simulink model "PID"  (R2022b)
settings: Solver=ode4  StartTime=0.0  StopTime=25  FixedStep=0.02  RelTol=1e-3  EnableMultiTasking=on
undefined symbols (not defined in the file): A3, B3, C2, DiscIntNeverNeededParam, rad, s
libraries: arduinolib x5, aerolibconvert2 x4, simulink_extras x1
settings Model: ExtModeTrigDuration=2  Creator=Ali  LastModifiedBy=Ali
settings SolverCC: AlgebraicLoopSolver=TrustRegion
settings OptimizationCC: EnhancedBackFolding=on  PassReuseOutputArgsAs=Individual arguments  ZeroExternalMemoryAtStartup=off  ZeroInternalMemoryAtStartup=off  MaxStackSize=64  OptimizeBlockOrder=speed  DifferentSizesBufferReuse=on  OptimizationCustomize=off  EfficientTunableParamExpr=on
settings DebuggingCC: ParameterTunabilityLossMsg=error  UnconnectedInputMsg=warning  UnconnectedOutputMsg=warning  UnconnectedLineMsg=warning  SFMachineParentedDataDiag=warning
settings HardwareCC: ProdBitPerInt=16  ProdBitPerPointer=16  ProdBitPerSizeT=16  ProdBitPerPtrDiffT=16  ProdLargestAtomicFloat=None  ProdWordSize=8  ProdHWDeviceType=Atmel->AVR
settings ModelReferenceCC: EnableRefExpFcnMdlSchedulingChecks=on
settings SFSimCC: MATLABDynamicMemAlloc=off
settings RTWCC: Description=Embedded Coder  SystemTargetFile=ert.tlc  HardwareBoard=Arduino Mega 2560  TLCOptions=-aInlineSetEventsForThisBaseRateFcn=TLC_FALSE -aSuppressMultiTaskScheduler=TLC_FALSE -aRateBasedStepFcn=1  TemplateMakefile=ert_default_tmf  Toolchain=Arduino AVR  BuildConfiguration=Faster Runs
settings CodeAppCC: ForceParamTrailComments=on  IgnoreCustomStorageClasses=off  OperatorAnnotations=on  SimulinkDataObjDesc=on  SFDataObjDesc=on  InsertBlockDesc=on
settings ERTTargetCC: SupportContinuousTime=on  SupportVariableSizeSignals=on  ExtModeStaticAllocSize=2048

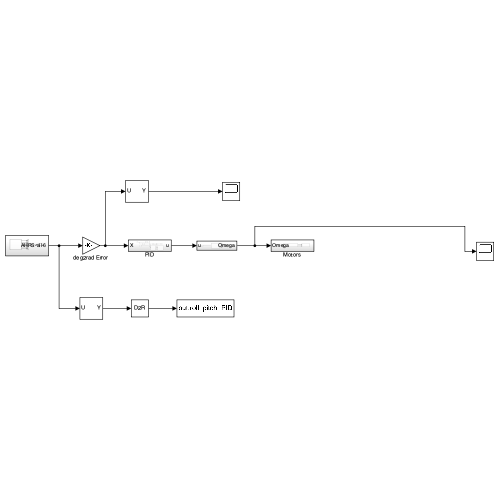
[thumbnail: Simulink's stored preview of the top-level diagram]
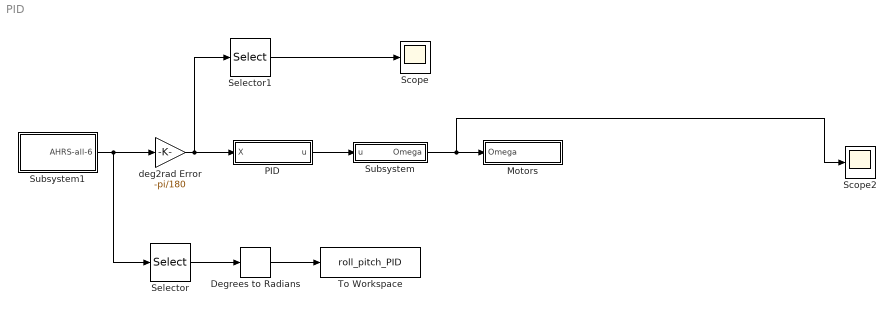
== system PID ==
  Degrees to Radians : simulink_extras/Transformations/Degrees to Radians
  Motors : Subsystem
  PID : Subsystem
  Scope : Scope
  Scope2 : Scope
  Selector : Selector  InputPortWidth=6  IndexOptions=Index vector (dialog)  Indices=[1 2 4 5]  OutputSizes=1
  Selector1 : Selector  InputPortWidth=6  IndexOptions=Index vector (dialog)  Indices=[1 2]  OutputSizes=1
  Subsystem : Subsystem
  Subsystem1 : Subsystem
  To Workspace : ToWorkspace  VariableName=roll_pitch_PID  SampleTime=-1
  deg2rad Error : Gain  Gain=-pi/180
  wires:
  Subsystem/1(Omega) -> Scope2/1, Motors/1(Omega)
  PID/1(u) -> Subsystem/1(u)
  Subsystem1/1(AHRS-all-6) -> Selector/1, deg2rad Error/1
  Selector/1 -> Degrees to Radians/1
  Degrees to Radians/1 -> To Workspace/1
  deg2rad Error/1 -> Selector1/1, PID/1(X)
  Selector1/1 -> Scope/1

== system PID/Motors ==
  Omega : Inport
  Arduino PWM1 : Subsystem  mask{Motor1=8, Motor2=9, Motor3=10, Motor4=11}
      mask prompts: Motor1 "Motor 1 Pin Number"; Motor2 "Motor 2 Pin Number"; Motor3 "Motor 3 Pin Number"; Motor4 "Motor 4 Pin Number"
  Convert To Duty Cycle : Subsystem
  Demux : Demux
  wires:
  Convert To Duty Cycle/4(duty_cycle4 (0-255)) -> Arduino PWM1/4(duty_cycle4 (0-255))
  Demux/4 -> Convert To Duty Cycle/4(Omega_Command4)
  Demux/3 -> Convert To Duty Cycle/3(Omega_Command3)
  Convert To Duty Cycle/2(duty_cycle2 (0-255)) -> Arduino PWM1/2(duty_cycle2 (0-255))
  Convert To Duty Cycle/1(duty_cycle1 (0-255)) -> Arduino PWM1/1(duty_cycle1 (0-255))
  Omega/1 -> Demux/1
  Demux/2 -> Convert To Duty Cycle/2(Omega_Command2)
  Demux/1 -> Convert To Duty Cycle/1(Omega_Command1)
  Convert To Duty Cycle/3(duty_cycle3 (0-255)) -> Arduino PWM1/3(duty_cycle3 (0-255))

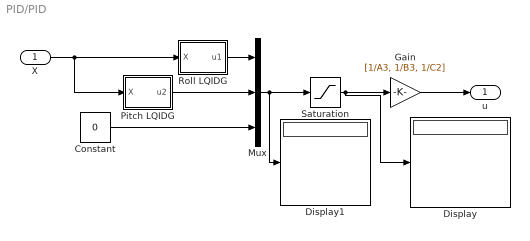
== system PID/PID ==
  X : Inport
  Constant : Constant  Value=0
  Display : Display
  Display1 : Display
  Gain : Gain  Gain=[1/A3, 1/B3, 1/C2]
  Mux : Mux  Inputs=3
  Pitch LQIDG : Subsystem
  Roll LQIDG : Subsystem
  Saturation : Saturate  UpperLimit=12  LowerLimit=-12
  u : Outport
  wires:
  Mux/1 -> Display1/1, Saturation/1
  Gain/1 -> u/1
  Saturation/1 -> Display/1, Gain/1
  Constant/1 -> Mux/3
  Pitch LQIDG/1(u2) -> Mux/2
  X/1 -> Pitch LQIDG/1(X), Roll LQIDG/1(X)
  Roll LQIDG/1(u1) -> Mux/1

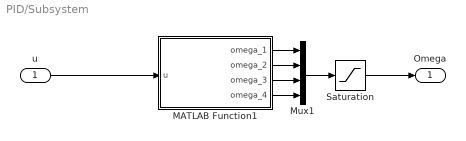
== system PID/Subsystem ==
  u : Inport
  MATLAB Function1 : MATLAB Function  TreatAsAtomicUnit=on
  Mux1 : Mux
  Saturation : Saturate  UpperLimit=6000/60*2*pi  LowerLimit=1000/60*2*pi
  Omega : Outport
  wires:
  MATLAB Function1/1(omega_1) -> Mux1/1
  MATLAB Function1/2(omega_2) -> Mux1/2
  MATLAB Function1/4(omega_4) -> Mux1/4
  Mux1/1 -> Saturation/1
  MATLAB Function1/3(omega_3) -> Mux1/3
  Saturation/1 -> Omega/1
  u/1 -> MATLAB Function1/1(u)

== system PID/Subsystem1 ==
  AHRS : Subsystem
  Mux : Mux  Inputs=6
  AHRS-all-6 : Outport
  wires:
  Mux/1 -> AHRS-all-6/1
  AHRS/4(roll_rate) -> Mux/4
  AHRS/2(theta) -> Mux/2
  AHRS/6(yaw_rate) -> Mux/6
  AHRS/1(phi) -> Mux/1
  AHRS/5(pitch_rate) -> Mux/5
  AHRS/3(psi) -> Mux/3

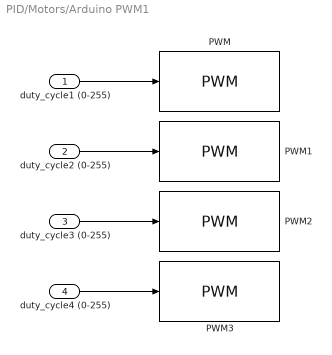
== system PID/Motors/Arduino PWM1 ==
  duty_cycle1 (0-255) : Inport
  duty_cycle2 (0-255) : Inport  Port=2
  duty_cycle3 (0-255) : Inport  Port=3
  duty_cycle4 (0-255) : Inport  Port=4
  PWM : arduinolib/PWM  pinNumber=8  frequencyType=Default  desiredFrequency=490.2  achievableFrequency=490.2
  PWM1 : arduinolib/PWM  pinNumber=9  frequencyType=Default  desiredFrequency=490.2  achievableFrequency=490.2
  PWM2 : arduinolib/PWM  pinNumber=10  frequencyType=Default  desiredFrequency=490.2  achievableFrequency=490.2
  PWM3 : arduinolib/PWM  pinNumber=11  frequencyType=Default  desiredFrequency=490.2  achievableFrequency=490.2
  wires:
  duty_cycle1 (0-255)/1 -> PWM/1
  duty_cycle2 (0-255)/1 -> PWM1/1
  duty_cycle3 (0-255)/1 -> PWM2/1
  duty_cycle4 (0-255)/1 -> PWM3/1

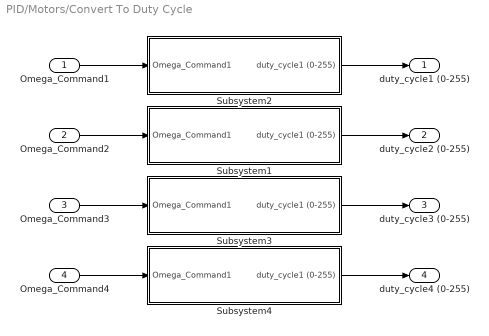
== system PID/Motors/Convert To Duty Cycle ==
  Omega_Command1 : Inport
  Omega_Command2 : Inport  Port=2
  Omega_Command3 : Inport  Port=3
  Omega_Command4 : Inport  Port=4
  Subsystem1 : Subsystem
  Subsystem2 : Subsystem
  Subsystem3 : Subsystem
  Subsystem4 : Subsystem
  duty_cycle1 (0-255) : Outport
  duty_cycle2 (0-255) : Outport  Port=2
  duty_cycle3 (0-255) : Outport  Port=3
  duty_cycle4 (0-255) : Outport  Port=4
  wires:
  Subsystem1/1(duty_cycle1 (0-255)) -> duty_cycle2 (0-255)/1
  Subsystem3/1(duty_cycle1 (0-255)) -> duty_cycle3 (0-255)/1
  Subsystem4/1(duty_cycle1 (0-255)) -> duty_cycle4 (0-255)/1
  Subsystem2/1(duty_cycle1 (0-255)) -> duty_cycle1 (0-255)/1
  Omega_Command1/1 -> Subsystem2/1(Omega_Command1)
  Omega_Command4/1 -> Subsystem4/1(Omega_Command1)
  Omega_Command3/1 -> Subsystem3/1(Omega_Command1)
  Omega_Command2/1 -> Subsystem1/1(Omega_Command1)

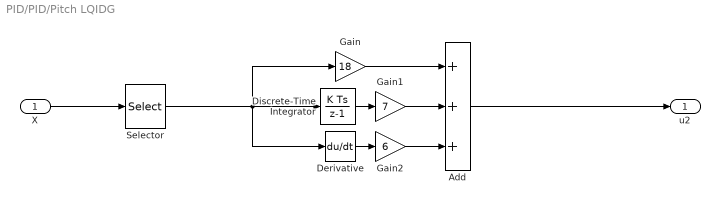
== system PID/PID/Pitch LQIDG ==
  X : Inport
  Add : Sum  Inputs=+++
  Derivative : Derivative
  Discrete-Time Integrator : DiscreteIntegrator  SampleTime=-1  ICPrevOutput=DiscIntNeverNeededParam  ICPrevScaledInput=DiscIntNeverNeededParam
  Gain : Gain  Gain=18
  Gain1 : Gain  Gain=7
  Gain2 : Gain  Gain=6
  Selector : Selector  InputPortWidth=6  IndexOptions=Index vector (dialog)  Indices=[2]  OutputSizes=1
  u2 : Outport
  wires:
  X/1 -> Selector/1
  Selector/1 -> Discrete-Time Integrator/1, Gain/1, Derivative/1
  Gain1/1 -> Add/2
  Gain2/1 -> Add/3
  Discrete-Time Integrator/1 -> Gain1/1
  Derivative/1 -> Gain2/1
  Gain/1 -> Add/1
  Add/1 -> u2/1

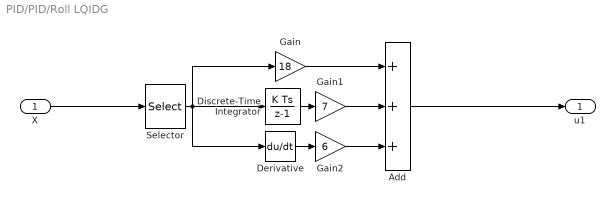
== system PID/PID/Roll LQIDG ==
  X : Inport
  Add : Sum  Inputs=+++
  Derivative : Derivative
  Discrete-Time Integrator : DiscreteIntegrator  SampleTime=-1  ICPrevOutput=DiscIntNeverNeededParam  ICPrevScaledInput=DiscIntNeverNeededParam
  Gain : Gain  Gain=18
  Gain1 : Gain  Gain=7
  Gain2 : Gain  Gain=6
  Selector : Selector  InputPortWidth=6  IndexOptions=Index vector (dialog)  Indices=[1]  OutputSizes=1
  u1 : Outport
  wires:
  X/1 -> Selector/1
  Selector/1 -> Discrete-Time Integrator/1, Derivative/1, Gain/1
  Gain/1 -> Add/1
  Discrete-Time Integrator/1 -> Gain1/1
  Gain1/1 -> Add/2
  Gain2/1 -> Add/3
  Derivative/1 -> Gain2/1
  Add/1 -> u1/1

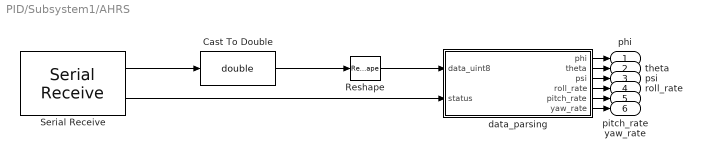
== system PID/Subsystem1/AHRS ==
  Cast To Double : DataTypeConversion  OutDataTypeStr=double  SaturateOnIntegerOverflow=off  RndMeth=Floor
  Reshape : Reshape
  Serial Receive : arduinolib/Serial Receive  isARMArch=off  portNumber=1  DataType=uint8  Datalength=32  SampleTime=0.02  showOutStatus=on  blockPlatform=arduino
  data_parsing : MATLAB Function  TreatAsAtomicUnit=on
  phi : Outport
  theta : Outport  Port=2
  psi : Outport  Port=3
  roll_rate : Outport  Port=4
  pitch_rate : Outport  Port=5
  yaw_rate : Outport  Port=6
  wires:
  data_parsing/2(theta) -> theta/1
  data_parsing/3(psi) -> psi/1
  data_parsing/4(roll_rate) -> roll_rate/1
  Reshape/1 -> data_parsing/1(data_uint8)
  data_parsing/1(phi) -> phi/1
  data_parsing/5(pitch_rate) -> pitch_rate/1
  Serial Receive/2 -> data_parsing/2(status)
  data_parsing/6(yaw_rate) -> yaw_rate/1
  Cast To Double/1 -> Reshape/1
  Serial Receive/1 -> Cast To Double/1

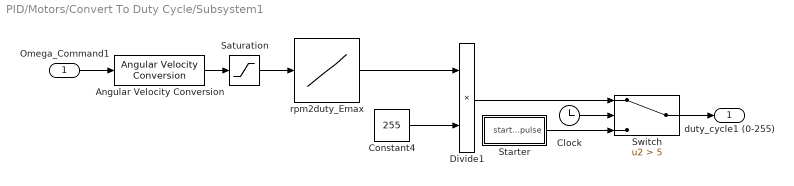
== system PID/Motors/Convert To Duty Cycle/Subsystem1 ==
  Omega_Command1 : Inport
  Angular Velocity Conversion : aerolibconvert2/Angular Velocity Conversion  IU=rad/s  OU=rpm
  Clock : Clock
  Constant4 : Constant  Value=255
  Divide1 : Product  Inputs=**
  Saturation : Saturate  UpperLimit=6000  LowerLimit=1300
  Starter : Subsystem
  Switch : Switch  Criteria=u2 > Threshold  Threshold=5  SaturateOnIntegerOverflow=off  InputSameDT=off
  rpm2duty_Emax : Lookup_n-D  NumberOfTableDimensions=1  BreakpointsForDimension1=|  Table=|  RndMeth=Simplest
      BreakpointsForDimension1=|
      | [1201
      | 2305
      | 3096
      | 3930
      | 4118
      | 4555
      | 5122
      | 5552
      | 5957
      | 6291
      | 6360]
      Table=|
      | [0.5
      | 0.55
      | 0.6
      | 0.65
      | 0.7
      | 0.75
      | 0.8
      | 0.85
      | 0.9
      | 0.95
      | 1]
  duty_cycle1 (0-255) : Outport
  wires:
  Divide1/1 -> Switch/1
  Switch/1 -> duty_cycle1 (0-255)/1
  Clock/1 -> Switch/2
  Starter/1(start_pulse) -> Switch/3
  Angular Velocity Conversion/1 -> Saturation/1
  Constant4/1 -> Divide1/2
  Omega_Command1/1 -> Angular Velocity Conversion/1
  rpm2duty_Emax/1 -> Divide1/1
  Saturation/1 -> rpm2duty_Emax/1

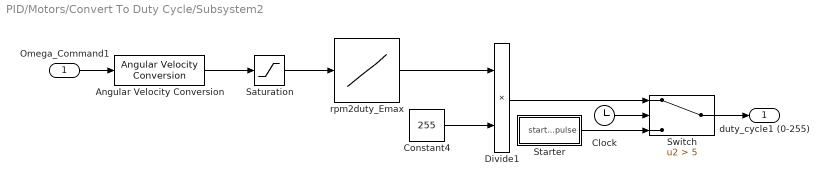
== system PID/Motors/Convert To Duty Cycle/Subsystem2 ==
  Omega_Command1 : Inport
  Angular Velocity Conversion : aerolibconvert2/Angular Velocity Conversion  IU=rad/s  OU=rpm
  Clock : Clock
  Constant4 : Constant  Value=255
  Divide1 : Product  Inputs=**
  Saturation : Saturate  UpperLimit=6000  LowerLimit=1300
  Starter : Subsystem
  Switch : Switch  Criteria=u2 > Threshold  Threshold=5  SaturateOnIntegerOverflow=off  InputSameDT=off
  rpm2duty_Emax : Lookup_n-D  NumberOfTableDimensions=1  BreakpointsForDimension1=|  Table=|  RndMeth=Simplest
      BreakpointsForDimension1=|
      | [1201
      | 2305
      | 3096
      | 3930
      | 4118
      | 4555
      | 5122
      | 5552
      | 5957
      | 6291
      | 6360]
      Table=|
      | [0.5
      | 0.55
      | 0.6
      | 0.65
      | 0.7
      | 0.75
      | 0.8
      | 0.85
      | 0.9
      | 0.95
      | 1]
  duty_cycle1 (0-255) : Outport
  wires:
  Omega_Command1/1 -> Angular Velocity Conversion/1
  Constant4/1 -> Divide1/2
  Angular Velocity Conversion/1 -> Saturation/1
  Starter/1(start_pulse) -> Switch/3
  Clock/1 -> Switch/2
  Switch/1 -> duty_cycle1 (0-255)/1
  Divide1/1 -> Switch/1
  rpm2duty_Emax/1 -> Divide1/1
  Saturation/1 -> rpm2duty_Emax/1

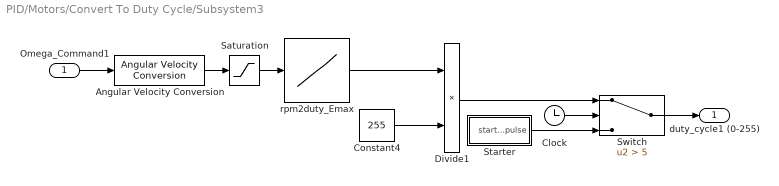
== system PID/Motors/Convert To Duty Cycle/Subsystem3 ==
  Omega_Command1 : Inport
  Angular Velocity Conversion : aerolibconvert2/Angular Velocity Conversion  IU=rad/s  OU=rpm
  Clock : Clock
  Constant4 : Constant  Value=255
  Divide1 : Product  Inputs=**
  Saturation : Saturate  UpperLimit=6000  LowerLimit=1300
  Starter : Subsystem
  Switch : Switch  Criteria=u2 > Threshold  Threshold=5  SaturateOnIntegerOverflow=off  InputSameDT=off
  rpm2duty_Emax : Lookup_n-D  NumberOfTableDimensions=1  BreakpointsForDimension1=|  Table=|  RndMeth=Simplest
      BreakpointsForDimension1=|
      | [1201
      | 2305
      | 3096
      | 3930
      | 4118
      | 4555
      | 5122
      | 5552
      | 5957
      | 6291
      | 6360]
      Table=|
      | [0.5
      | 0.55
      | 0.6
      | 0.65
      | 0.7
      | 0.75
      | 0.8
      | 0.85
      | 0.9
      | 0.95
      | 1]
  duty_cycle1 (0-255) : Outport
  wires:
  Omega_Command1/1 -> Angular Velocity Conversion/1
  Constant4/1 -> Divide1/2
  Angular Velocity Conversion/1 -> Saturation/1
  Starter/1(start_pulse) -> Switch/3
  Clock/1 -> Switch/2
  Switch/1 -> duty_cycle1 (0-255)/1
  Divide1/1 -> Switch/1
  rpm2duty_Emax/1 -> Divide1/1
  Saturation/1 -> rpm2duty_Emax/1

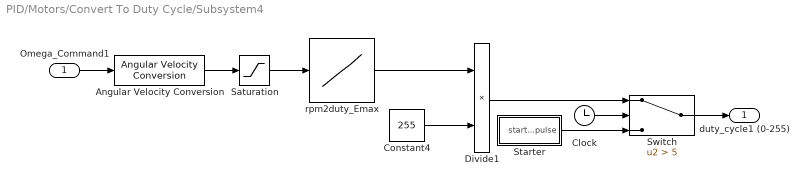
== system PID/Motors/Convert To Duty Cycle/Subsystem4 ==
  Omega_Command1 : Inport
  Angular Velocity Conversion : aerolibconvert2/Angular Velocity Conversion  IU=rad/s  OU=rpm
  Clock : Clock
  Constant4 : Constant  Value=255
  Divide1 : Product  Inputs=**
  Saturation : Saturate  UpperLimit=6000  LowerLimit=1300
  Starter : Subsystem
  Switch : Switch  Criteria=u2 > Threshold  Threshold=5  SaturateOnIntegerOverflow=off  InputSameDT=off
  rpm2duty_Emax : Lookup_n-D  NumberOfTableDimensions=1  BreakpointsForDimension1=|  Table=|  RndMeth=Simplest
      BreakpointsForDimension1=|
      | [1201
      | 2305
      | 3096
      | 3930
      | 4118
      | 4555
      | 5122
      | 5552
      | 5957
      | 6291
      | 6360]
      Table=|
      | [0.5
      | 0.55
      | 0.6
      | 0.65
      | 0.7
      | 0.75
      | 0.8
      | 0.85
      | 0.9
      | 0.95
      | 1]
  duty_cycle1 (0-255) : Outport
  wires:
  Divide1/1 -> Switch/1
  Switch/1 -> duty_cycle1 (0-255)/1
  Clock/1 -> Switch/2
  Starter/1(start_pulse) -> Switch/3
  Angular Velocity Conversion/1 -> Saturation/1
  Constant4/1 -> Divide1/2
  Omega_Command1/1 -> Angular Velocity Conversion/1
  rpm2duty_Emax/1 -> Divide1/1
  Saturation/1 -> rpm2duty_Emax/1

== system PID/Motors/Convert To Duty Cycle/Subsystem1/Starter ==
  Add : Sum
  Step : Step  After=140
  Step1 : Step  Time=2  After=-30
  start_pulse : Outport
  wires:
  Add/1 -> start_pulse/1
  Step/1 -> Add/1
  Step1/1 -> Add/2

== system PID/Motors/Convert To Duty Cycle/Subsystem2/Starter ==
  Add : Sum
  Step : Step  After=140
  Step1 : Step  Time=2  After=-30
  start_pulse : Outport
  wires:
  Add/1 -> start_pulse/1
  Step/1 -> Add/1
  Step1/1 -> Add/2

== system PID/Motors/Convert To Duty Cycle/Subsystem3/Starter ==
  Add : Sum
  Step : Step  After=140
  Step1 : Step  Time=2  After=-30
  start_pulse : Outport
  wires:
  Add/1 -> start_pulse/1
  Step/1 -> Add/1
  Step1/1 -> Add/2

== system PID/Motors/Convert To Duty Cycle/Subsystem4/Starter ==
  Add : Sum
  Step : Step  After=140
  Step1 : Step  Time=2  After=-30
  start_pulse : Outport
  wires:
  Add/1 -> start_pulse/1
  Step/1 -> Add/1
  Step1/1 -> Add/2

== matlab function PID/Subsystem/MATLAB Function1 ==
  data: u input size=3; omega_1 output size=1; omega_2 output size=1; omega_3 output size=1; omega_4 output size=1
function [omega_1, omega_2, omega_3, omega_4] = fcn(u)
u1 = u(1);
u2 = u(2);
u3 = u(3);
% control effort
u4 = ones(1, length(u1)) * 4 * rpm2rad_sec(2050)^2;
% calculate omega
if (u4 + u3 + 2 * u2) / 4 > 0
    omega_1 = sqrt((u4 + u3 + 2 * u2) / 4);
else
    omega_1 = 0;
end
if (u4 + u3 - 2 * u2) / 4 > 0
    omega_3 = sqrt((u4 + u3 - 2 * u2) / 4);
else
    omega_3 = 0;
end
if (u4 - u3 + 2 * u1) / 4 > 0
    omega_2 = sqrt((u4 - u3 + 2 * u1) / 4);
else
    omega_2 = 0;
end
if (u4 - u3 - 2 * u1) / 4 > 0
    omega_4 = sqrt((u4 - u3 - 2 * u1) / 4);
else
    omega_4 = 0;
end
end
%% functions
% rpm to rad/sec
function rad = rpm2rad_sec(rpm)
rad = rpm / 60 * 2 * pi;
end

== matlab function PID/Subsystem1/AHRS/data_parsing ==
  data: phi output size=1; data_uint8 input size=32; theta output size=1; psi output size=1; roll_rate output size=1; pitch_rate output size=1; yaw_rate output size=1; status input
function [phi,theta,psi,roll_rate,pitch_rate,yaw_rate] = fcn(data_uint8, status)
persistent stepp check_sum...
    phi_p theta_p psi_p roll_rate_p pitch_rate_p yaw_rate_p...
    phi_last theta_last psi_last roll_rate_last pitch_rate_last yaw_rate_last;
%% Initialize
if isempty(stepp)
    stepp=0;
    check_sum=0;
    phi_p=0;
    theta_p=0;
    psi_p=0;
    roll_rate_p=0;
    pitch_rate_p=0;
    yaw_rate_p=0;
    phi_last=0;
    theta_last=0;
    psi_last=0;
    roll_rate_last=0;
    pitch_rate_last=0;
    yaw_rate_last=0;
end
angle_scale=.0109863;  % 1/91.0222
rate_scale=1/16;
%% Check Each Byte
if status
    for i = 1:length(data_uint8)
        if (data_uint8(i)==115 && stepp==0)
            stepp=1;
            check_sum=data_uint8(i);
        elseif(stepp==1 && data_uint8(i)==110)
            stepp=stepp+1;
            check_sum=check_sum+data_uint8(i);
        elseif(stepp==2 && data_uint8(i)==112)
            stepp=stepp+1;
            check_sum=check_sum+data_uint8(i);
        elseif(stepp==3 && data_uint8(i)==212)
            stepp=stepp+1;
            check_sum=check_sum+data_uint8(i);
        elseif(stepp==4 && data_uint8(i)==112)
            stepp=stepp+1;
            check_sum=check_sum+data_uint8(i);
        elseif(stepp==5)
            phi_p=data_uint8(i)*256;
            stepp=stepp+1;
            check_sum=check_sum+data_uint8(i);
        elseif(stepp==6)
            phi_p=phi_p+data_uint8(i);
            stepp=stepp+1;
            check_sum=check_sum+data_uint8(i);
        elseif(stepp==7)
            theta_p=data_uint8(i)*256;
            stepp=stepp+1;
            check_sum=check_sum+data_uint8(i);
        elseif(stepp==8)
            theta_p=theta_p+data_uint8(i);
            stepp=stepp+1;
            check_sum=check_sum+data_uint8(i);
        elseif(stepp==9)
            psi_p=data_uint8(i)*256;
            stepp=stepp+1;
            check_sum=check_sum+data_uint8(i);
        elseif(stepp==10)
            psi_p=psi_p+data_uint8(i);
            stepp=stepp+1;
            check_sum=check_sum+data_uint8(i);
        elseif(stepp==11 || stepp==12)
            if(data_uint8(i)==0)
                stepp=stepp+1;
            else
                stepp=0;
            end
        elseif(stepp==13)
            roll_rate_p=data_uint8(i)*256;
            stepp=stepp+1;
            check_sum=check_sum+data_uint8(i);
        elseif(stepp==14)
            roll_rate_p=roll_rate_p+data_uint8(i);
            stepp=stepp+1;
            check_sum=check_sum+data_uint8(i);
        elseif(stepp==15)
            pitch_rate_p=data_uint8(i)*256;
            stepp=stepp+1;
            check_sum=check_sum+data_uint8(i);
        elseif(stepp==16)
            pitch_rate_p=pitch_rate_p+data_uint8(i);
            stepp=stepp+1;
            check_sum=check_sum+data_uint8(i);
        elseif(stepp==17)
            yaw_rate_p=data_uint8(i)*256;
            stepp=stepp+1;
            check_sum=check_sum+data_uint8(i);
        elseif(stepp==18)
            yaw_rate_p=yaw_rate_p+data_uint8(i);
            stepp=stepp+1;
            check_sum=check_sum+data_uint8(i);
        elseif(stepp==19 || stepp==20)
            if(data_uint8(i)==0)
                stepp=stepp+1;
            else
                stepp=0;
            end
        elseif(stepp==21 || stepp==22 || stepp==23 || stepp==24)
            stepp=stepp+1;
            check_sum=check_sum+data_uint8(i);
        elseif(stepp==25)
            if (floor(check_sum/256)==data_uint8(i))
                stepp=stepp+1;
            else
                stepp=0;
            end
        elseif(stepp==26)
            if(mod(check_sum,256)==data_uint8(i))
                phi_last=double(typecast(uint16(phi_p), 'int16'))*angle_scale;
                if mod(phi_last,360)>180
                    phi_last=mod(phi_last,360)-360;
                else
                    phi_last=mod(phi_last,360);
                end
                theta_last=double(typecast(uint16(theta_p), 'int16'))*angle_scale;
                if mod(theta_last,360)>180
                    theta_last=mod(theta_last,360)-360;
                else
                    theta_last=mod(theta_last,360);
                end
                psi_last=double(typecast(uint16(psi_p), 'int16'))*angle_scale;
                if mod(psi_last,360)>180
                    psi_last=mod(psi_last,360)-360;
                else
                    psi_last=mod(psi_last,360);
                end
                roll_rate_last=double(typecast(uint16(roll_rate_p), 'int16'))*rate_scale;
                if mod(roll_rate_last,360)>180
                    roll_rate_last=mod(roll_rate_last,360)-360;
                else
                    roll_rate_last=mod(roll_rate_last,360);
                end
                pitch_rate_last=double(typecast(uint16(pitch_rate_p), 'int16'))*rate_scale;
                if mod(pitch_rate_last,360)>180
                    pitch_rate_last=mod(pitch_rate_last,360)-360;
                else
                    pitch_rate_last=mod(pitch_rate_last,360);
                end
                yaw_rate_last=double(typecast(uint16(yaw_rate_p), 'int16'))*rate_scale;
                if mod(yaw_rate_last,360)>180
                    yaw_rate_last=mod(yaw_rate_last,360)-360;
                else
                    yaw_rate_last=mod(yaw_rate_last,360);
                end
            end
            stepp=0;
        end
    end
end

%% Assign Last True Data to Output
phi=phi_last;
theta=theta_last;
psi=psi_last;
roll_rate=roll_rate_last;
pitch_rate=pitch_rate_last;
yaw_rate=yaw_rate_last;
